simulink model "VOO_group11"  (R2023a)
settings: Solver=FixedStepAuto  StartTime=0.0  StopTime=10.0  FixedStep=1e-3  RelTol=1e-3  EnableMultiTasking=on
undefined symbols (not defined in the file): D10, D12, D2, D5, D7, D9, PTA2, PTB9, PTC3, PTC4, PTD0, PTD3
libraries: frdmk64flib x8
settings Model: ExtModeTrigDuration=5  Creator=faraa  LastModifiedBy=faraa
settings OptimizationCC: EnhancedBackFolding=on  PassReuseOutputArgsAs=Individual arguments  ZeroExternalMemoryAtStartup=off  ZeroInternalMemoryAtStartup=off  MaxStackSize=64  OptimizeBlockOrder=speed  DifferentSizesBufferReuse=on  OptimizationCustomize=off  EfficientTunableParamExpr=on
settings DebuggingCC: ParameterTunabilityLossMsg=error
settings HardwareCC: ProdBitPerPointer=32  ProdBitPerSizeT=32  ProdBitPerPtrDiffT=32  ProdLargestAtomicInteger=Long  ProdLargestAtomicFloat=Double  ProdWordSize=32  ProdHWDeviceType=ARM Compatible->ARM Cortex
settings SFSimCC: MATLABDynamicMemAlloc=off
settings RTWCC: Description=Embedded Coder  SystemTargetFile=ert.tlc  HardwareBoard=NXP FRDM-K64F  TLCOptions="-aInlineSetEventsForThisBaseRateFcn=TLC_FALSE -aSuppressMultiTaskScheduler=TLC_FALSE  -aRateBasedStepFcn=0"  TemplateMakefile=ert_default_tmf  Toolchain=GNU Tools for ARM Embedded Processors
settings CodeAppCC: ForceParamTrailComments=on  IgnoreCustomStorageClasses=off  OperatorAnnotations=on  SimulinkDataObjDesc=on  SFDataObjDesc=on  InsertBlockDesc=on
settings ERTTargetCC: ExtModeTransport=4  ExtModeMexFile=sendToCommService

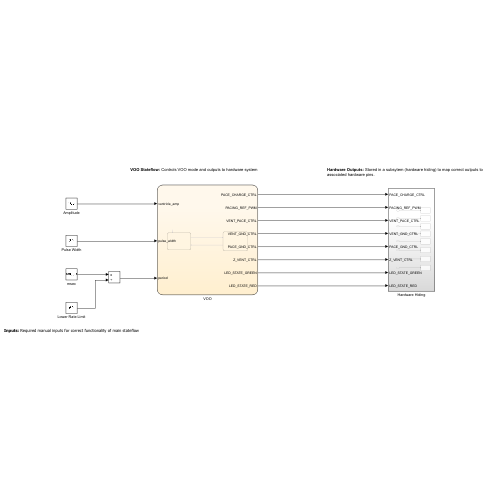
[thumbnail: Simulink's stored preview of the top-level diagram]
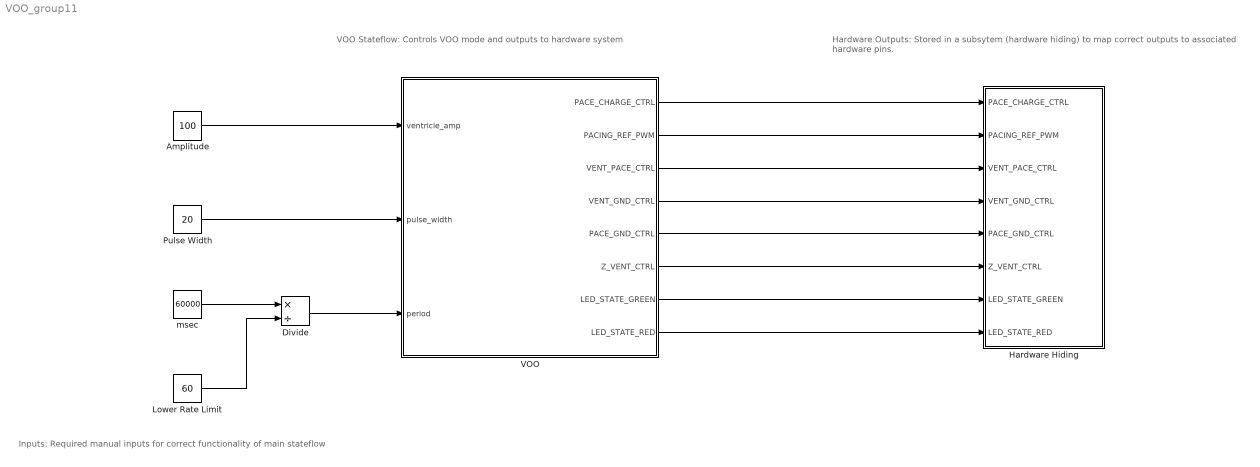
== system VOO_group11 ==
  note: Inputs: Required manual inputs for correct functionality of main stateflow
  note: VOO Stateflow: Controls VOO mode and outputs to hardware system
  note: Hardware Outputs: Stored in a subsytem (hardware hiding) to map correct outputs to associated hardware pins.
  Amplitude : Constant  Value=100
  Divide : Product  Inputs=*/
  Hardware Hiding : Subsystem
  Lower Rate Limit : Constant  Value=60
  Pulse Width : Constant  Value=20
  VOO : Stateflow chart  TreatAsAtomicUnit=on
  msec : Constant  Value=60000
  wires:
  Amplitude/1 -> VOO/1(ventricle_amp)
  Pulse Width/1 -> VOO/2(pulse_width)
  Divide/1 -> VOO/3(period)
  msec/1 -> Divide/1
  Lower Rate Limit/1 -> Divide/2
  VOO/1(PACE_CHARGE_CTRL) -> Hardware Hiding/1(PACE_CHARGE_CTRL)
  VOO/2(PACING_REF_PWM) -> Hardware Hiding/2(PACING_REF_PWM)
  VOO/3(VENT_PACE_CTRL) -> Hardware Hiding/3(VENT_PACE_CTRL)
  VOO/4(VENT_GND_CTRL) -> Hardware Hiding/4(VENT_GND_CTRL)
  VOO/5(PACE_GND_CTRL) -> Hardware Hiding/5(PACE_GND_CTRL)
  VOO/6(Z_VENT_CTRL) -> Hardware Hiding/6(Z_VENT_CTRL)
  VOO/7(LED_STATE_GREEN) -> Hardware Hiding/7(LED_STATE_GREEN)
  VOO/8(LED_STATE_RED) -> Hardware Hiding/8(LED_STATE_RED)

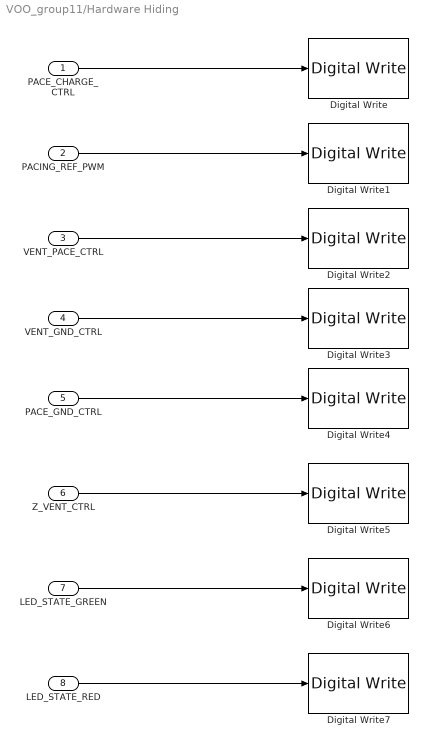
== system VOO_group11/Hardware Hiding ==
  PACE_CHARGE_CTRL : Inport
  PACING_REF_PWM : Inport  Port=2
  VENT_PACE_CTRL : Inport  Port=3
  VENT_GND_CTRL : Inport  Port=4
  PACE_GND_CTRL : Inport  Port=5
  Z_VENT_CTRL : Inport  Port=6
  LED_STATE_GREEN : Inport  Port=7
  LED_STATE_RED : Inport  Port=8
  Digital Write : frdmk64flib/Digital Write  Whichpin=PTB9 (D2)
  Digital Write1 : frdmk64flib/Digital Write  Whichpin=PTA2 (D5)
  Digital Write2 : frdmk64flib/Digital Write  Whichpin=PTC4 (D9)
  Digital Write3 : frdmk64flib/Digital Write  Whichpin=PTD3 (D12)
  Digital Write4 : frdmk64flib/Digital Write  Whichpin=PTD0 (D10)
  Digital Write5 : frdmk64flib/Digital Write  Whichpin=PTC3 (D7)
  Digital Write6 : frdmk64flib/Digital Write  Whichpin=GREEN_LED
  Digital Write7 : frdmk64flib/Digital Write  Whichpin=RED_LED
  wires:
  PACE_CHARGE_CTRL/1 -> Digital Write/1
  PACING_REF_PWM/1 -> Digital Write1/1
  VENT_PACE_CTRL/1 -> Digital Write2/1
  VENT_GND_CTRL/1 -> Digital Write3/1
  PACE_GND_CTRL/1 -> Digital Write4/1
  Z_VENT_CTRL/1 -> Digital Write5/1
  LED_STATE_GREEN/1 -> Digital Write6/1
  LED_STATE_RED/1 -> Digital Write7/1

== stateflow chart VOO_group11/VOO ==
  note: Charging: State to Charge C22 and discharge C21
      | and trigger LED indicators
  note: Pacing: Discharges C22 and charges C21
      | and triggers LED indicators
  state Pacing
    entry:
    PACING_REF_PWM = ventricle_amp;
    PACE_CHARGE_CTRL=0;
    VENT_PACE_CTRL= 1;
    VENT_GND_CTRL= 0;
    PACE_GND_CTRL=1;
    Z_VENT_CTRL=0;
    LED_STATE_RED=false;
    LED_STATE_GREEN=true;
  state Charging
    entry:
    PACING_REF_PWM = ventricle_amp;
    PACE_CHARGE_CTRL = 1;
    VENT_PACE_CTRL = 0;
    VENT_GND_CTRL = 1;
    PACE_GND_CTRL = 0;
    Z_VENT_CTRL = 0;
    LED_STATE_RED=true;
    LED_STATE_GREEN=false;
  (default) -> Charging
  Charging -> Pacing : [after(period-pulse_width,msec)]
  Pacing -> Charging : [after(pulse_width,msec)]
  data: ventricle_amp input; pulse_width input; period input; PACE_CHARGE_CTRL output; PACING_REF_PWM output; VENT_PACE_CTRL output; VENT_GND_CTRL output; PACE_GND_CTRL output; Z_VENT_CTRL output; LED_STATE_GREEN output; LED_STATE_RED output
